simulink model "ex7"  (Simulink 6.0)
settings: Solver=VariableStepDiscrete  StartTime=0.0  StopTime=SimulationTime  RelTol=1e-3
libraries: commutil2 x4, commsink2 x2, commfilt2 x2, commdigbbndpm2 x2, commchan2 x1, commrandsrc2 x1
settings Model: LastModifiedBy=lxy

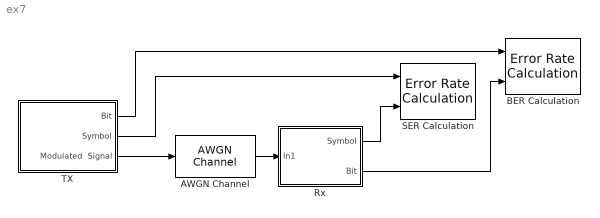
== system ex7 ==
  AWGN Channel : commchan2/AWGN Channel  seed=123456  noiseMode="Signal to noise ratio  (SNR)"  EbNodB=10  EsNodB=10  SNRdB=SNR  bitsPerSym=1  Ps=1  Tsym=1  variance=1
  BER Calculation : commsink2/Error Rate Calculation  N=0  st_delay=0  cp_mode=Entire frame  subframe=[]  PMode=Workspace  WsName=BER  RsMode2=off  stop=off  numErr=100  maxBits=1e6
  Rx : Subsystem
  SER Calculation : commsink2/Error Rate Calculation  N=0  st_delay=0  cp_mode=Entire frame  subframe=[]  PMode=Workspace  WsName=SER  RsMode2=off  stop=off  numErr=100  maxBits=1e6
  TX : Subsystem
  wires:
  TX/3(Modulated  Signal) -> AWGN Channel/1
  AWGN Channel/1 -> Rx/1(In1)
  TX/2(Symbol) -> SER Calculation/1
  Rx/1(Symbol) -> SER Calculation/2
  TX/1(Bit) -> BER Calculation/1
  Rx/2(Bit) -> BER Calculation/2

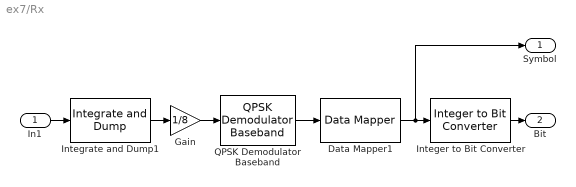
== system ex7/Rx ==
  In1 : Inport  Port=1  LatchInput=off
  Data Mapper1 : commutil2/Data Mapper  MapMode=Gray to Binary  M=4  MapVec=[0 1 3 2 7 6 4 5]
  Gain : Gain  Gain=1/8
  Integer to Bit Converter : commutil2/Integer to Bit Converter  nbits=2
  Integrate and Dump1 : commfilt2/Integrate and Dump  obssamples=8  offsetsamples=0  nodump=off
  QPSK Demodulator Baseband : commdigbbndpm2/QPSK Demodulator Baseband  OutType=Integer  Dec=Binary  Ph=0  numSamp=1
  Symbol : Outport
  Bit : Outport  Port=2
  wires:
  Integrate and Dump1/1 -> Gain/1
  Integer to Bit Converter/1 -> Bit/1
  Data Mapper1/1 -> Integer to Bit Converter/1, Symbol/1
  QPSK Demodulator Baseband/1 -> Data Mapper1/1
  In1/1 -> Integrate and Dump1/1
  Gain/1 -> QPSK Demodulator Baseband/1

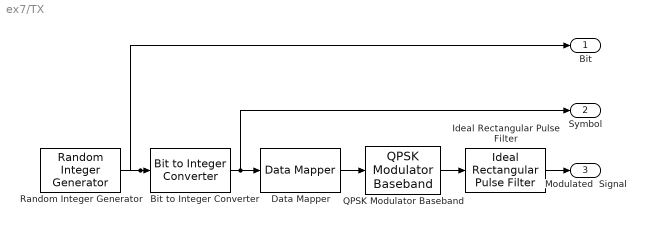
== system ex7/TX ==
  Bit to Integer Converter : commutil2/Bit to Integer Converter  nbits=2
  Data Mapper : commutil2/Data Mapper  MapMode=Binary to Gray  M=4  MapVec=[0 1 3 2 7 6 4 5]
  Ideal Rectangular Pulse Filter : commfilt2/Ideal Rectangular Pulse Filter  pulseLen=8  pulseDelay=0  sampMode=Frame-based  normCheck=off  normMode=Energy per pulse  filterGain=1
  QPSK Modulator Baseband : commdigbbndpm2/QPSK Modulator Baseband  InType=Integer  Enc=Binary  Ph=0  numSamp=1
  Random Integer Generator : commrandsrc2/Random Integer Generator  mul=2  seed=37  Ts=1/400000  frameBased=on  sampPerFrame=400000  orient=off
  Bit : Outport
  Symbol : Outport  Port=2
  Modulated  Signal : Outport  Port=3
  wires:
  Ideal Rectangular Pulse Filter/1 -> Modulated  Signal/1
  Random Integer Generator/1 -> Bit to Integer Converter/1, Bit/1
  Bit to Integer Converter/1 -> Data Mapper/1, Symbol/1
  Data Mapper/1 -> QPSK Modulator Baseband/1
  QPSK Modulator Baseband/1 -> Ideal Rectangular Pulse Filter/1
